simulink model "Practica1"  (R2020b)
settings: Solver=VariableStepAuto  StartTime=0.0  StopTime=1.2  RelTol=1e-20
libraries: simulink x1
settings Model: Creator=César  LastModifiedBy=cesar
settings SolverCC: ZeroCrossControl=DisableAll

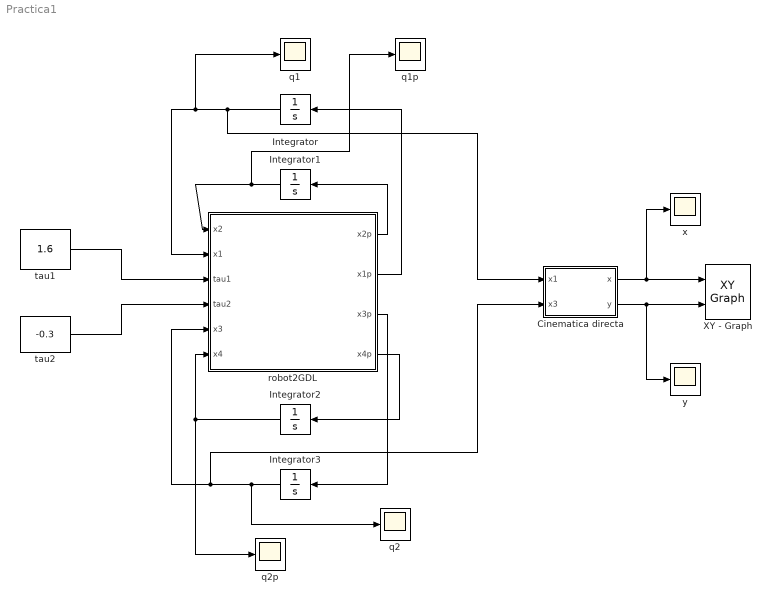
== system Practica1 ==
  Cinematica directa : MATLAB Function  TreatAsAtomicUnit=on
  Integrator{,1..3} (4 alike) : Integrator
  XY - Graph : simulink/Sinks/XY Graph  xmin=-0.4  xmax=0.4  ymin=-0.4  ymax=0.4  st=-1
  q1 : Scope
  q1p : Scope
  q2 : Scope
  q2p : Scope
  robot2GDL : MATLAB Function  TreatAsAtomicUnit=on
  tau1 : Constant  Value=1.6
  tau2 : Constant  Value=-0.3
  x : Scope
  y : Scope
  wires:
  robot2GDL/4(x4p) -> Integrator2/1
  Integrator2/1 -> q2p/1, robot2GDL/6(x4)
  robot2GDL/1(x2p) -> Integrator1/1
  Integrator1/1 -> q1p/1, robot2GDL/1(x2)
  robot2GDL/2(x1p) -> Integrator/1
  Integrator/1 -> q1/1, robot2GDL/2(x1), Cinematica directa/1(x1)
  robot2GDL/3(x3p) -> Integrator3/1
  Integrator3/1 -> q2/1, robot2GDL/5(x3), Cinematica directa/2(x3)
  tau2/1 -> robot2GDL/4(tau2)
  tau1/1 -> robot2GDL/3(tau1)
  Cinematica directa/1(x) -> XY - Graph/1, x/1
  Cinematica directa/2(y) -> XY - Graph/2, y/1

== matlab function Practica1/Cinematica directa ==
  data: x output; x1 input; y output; x3 input
function [x, y] = fcn(x1, x3)

l1 = 0.1933;   % m (metros)
l2 = 0.1458;   % m (metros)

x = l1*sin(x1) + l2*sin(x1 + x3);
y = -l1*cos(x1) - l2*cos(x1 + x3);

== matlab function Practica1/robot2GDL ==
  data: x2 input; x2p output; x1 input; x1p output; tau1 input; tau2 input; x3 input; x4 input; x3p output; x4p output
function [x2p,x1p,x3p,x4p] = fcn(x2,x1,tau1,tau2,x3,x4)
%Parámetros del sistema
m1 = 0.4272;   % masa kg
m2 = 0.3442;   % masa kg
I1 = 0.0036;   % kg*m^2 (momento de inercia)
I2 = 0.0021;   % kg*m^2 (momento de inercia)
l1 = 0.1933;   % m (metros)
l2 = 0.1458;   % m (metros)
lc1 = 0.0741;  % m (metros)
lc2 = 0.04849; % m (metros)
g = 9.81;     % m/s^2 (gravedad de la tierra)
%Modelo del sistema
M11 = m1*lc1^2 + m2*l1^2 + m2*lc2^2 + 2*m2*l1*lc2*cos(x3) + I1 + I2;
M12 = m2*lc2^2 + m2*l1*lc2*cos(x3) + I2;
M21 = m2*lc2^2 + m2*l1*lc2*cos(x3) + I2;
M22 = m2*lc2^2 + I2;
C11 = -m2*l1*lc2*sin(x3)*x4;
C12 = m2*l1*lc2*sin(x3)*(x2 + x4);
C21 = m2*l1*lc2*sin(x3)*x2;
C22 = 0;
g1 = (m1*lc1 + m2*l1)*g*sin(x1) + m2*lc2*g*sin(x1 + x3);
g2 = m2*lc2*g*sin(x1 + x3);

delta4 = M11*M22 - M12*M21;
delta5 = tau1 - C11*x2 - C12*x4 - g1;
delta6 = tau2 - C21*x2 - C22*x4 - g2;
%Modelo del sistema en representación de estado
x1p = x2;
x2p = (M22*delta5 - M12*delta6)/delta4;
x3p = x4;
x4p = (-M21*delta5 + M11*delta6)/delta4;
